simulink model "R2"  (R2016a)
settings: Solver=VariableStepAuto  StartTime=0.0  StopTime=15  MaxStep=0.01  RelTol=1e-3
values from neighbouring files (symbols this model uses):
  A = [0, 1, 0, 0 ... (first row only)    [Data.m]
  B = [0 ; 0; 0; 1]    [Data.m]
  K = acker (A, B, P)    [Data.m]
  l = 50    [Data.m]
settings Model: Creator=NAD  LastModifiedBy=NAD

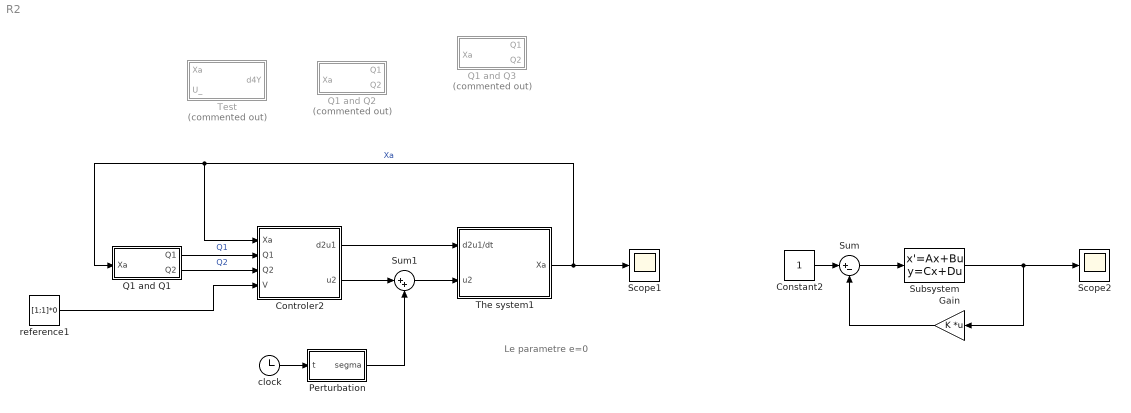
== system R2 ==
  note: Le parametre e=0
  Constant2 : Constant
  Controler2 : MATLAB Function  TreatAsAtomicUnit=on
  Gain : Gain  Gain=K  Multiplication=Matrix(K*u) (u vector)
  Perturbation : MATLAB Function  TreatAsAtomicUnit=on
  Q1 and Q1 : Subsystem
  Q1 and Q2 : Subsystem  Commented=on
  Q1 and Q3 : Subsystem  Commented=on
  Scope1 : Scope
  Scope2 : Scope
  Subsystem : StateSpace  A=A  B=B  C=eye(4)  D=[0 0 0 0 ]'  X0=0
  Sum : Sum  Inputs=|+-
  Sum1 : Sum  Inputs=|++
  Test : MATLAB Function  Commented=on  TreatAsAtomicUnit=on
  The system1 : Subsystem
  clock : Clock
  reference1 : Constant  Value=[1;1]*0
  wires:
  Subsystem/1 -> Scope2/1, Gain/1
  Sum/1 -> Subsystem/1
  Gain/1 -> Sum/2
  Constant2/1 -> Sum/1
  The system1/1(Xa) -> Q1 and Q1/1(Xa), Controler2/1(Xa), Scope1/1  "Xa"
  reference1/1 -> Controler2/4(V)
  Q1 and Q1/1(Q1) -> Controler2/2(Q1)  "Q1"
  Q1 and Q1/2(Q2) -> Controler2/3(Q2)  "Q2"
  Controler2/1(d2u1) -> The system1/1(d2u1/dt)
  Controler2/2(u2) -> Sum1/1
  Sum1/1 -> The system1/2(u2)
  clock/1 -> Perturbation/1(t)
  Perturbation/1(segma) -> Sum1/2

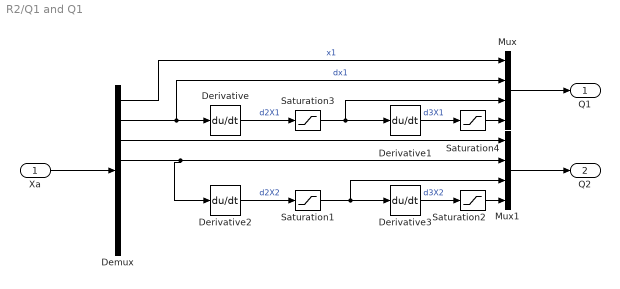
== system R2/Q1 and Q1 ==
  Xa : Inport
  Demux : Demux  Outputs=8
  Derivative{,1..3} (4 alike) : Derivative
  Mux : Mux
  Mux1 : Mux
  Saturation{1..4} (4 alike) : Saturate  UpperLimit=l  LowerLimit=-l  ZeroCross=off
  Q1 : Outport
  Q2 : Outport  Port=2
  wires:
  Mux1/1 -> Q2/1
  Mux/1 -> Q1/1
  Demux/3 -> Mux1/1
  Derivative1/1 -> Saturation4/1  "d3X1"
  Demux/1 -> Mux/1  "x1"
  Xa/1 -> Demux/1
  Derivative3/1 -> Saturation2/1  "d3X2"
  Demux/4 -> Derivative2/1, Mux1/2
  Demux/2 -> Mux/2, Derivative/1  "dx1"
  Saturation4/1 -> Mux/4
  Saturation2/1 -> Mux1/4
  Derivative2/1 -> Saturation1/1  "d2X2"
  Derivative/1 -> Saturation3/1  "d2X1"
  Saturation3/1 -> Mux/3, Derivative1/1
  Saturation1/1 -> Derivative3/1, Mux1/3

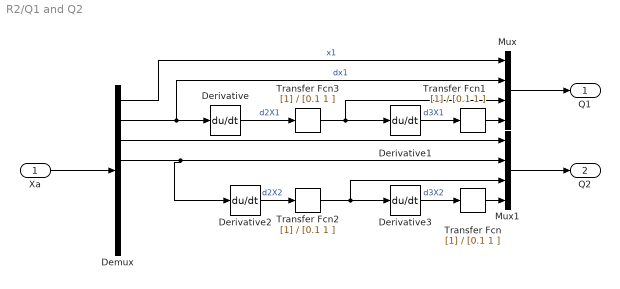
== system R2/Q1 and Q2 ==
  Xa : Inport
  Demux : Demux  Outputs=8
  Derivative{,1..3} (4 alike) : Derivative
  Mux : Mux
  Mux1 : Mux
  Transfer Fcn{,1..3} (4 alike) : TransferFcn  Denominator=[0.1 1 ]
  Q1 : Outport
  Q2 : Outport  Port=2
  wires:
  Mux1/1 -> Q2/1
  Mux/1 -> Q1/1
  Demux/3 -> Mux1/1
  Derivative1/1 -> Transfer Fcn1/1  "d3X1"
  Demux/1 -> Mux/1  "x1"
  Xa/1 -> Demux/1
  Derivative3/1 -> Transfer Fcn/1  "d3X2"
  Demux/4 -> Derivative2/1, Mux1/2
  Demux/2 -> Mux/2, Derivative/1  "dx1"
  Transfer Fcn1/1 -> Mux/4
  Transfer Fcn/1 -> Mux1/4
  Derivative2/1 -> Transfer Fcn2/1  "d2X2"
  Derivative/1 -> Transfer Fcn3/1  "d2X1"
  Transfer Fcn3/1 -> Mux/3, Derivative1/1
  Transfer Fcn2/1 -> Derivative3/1, Mux1/3

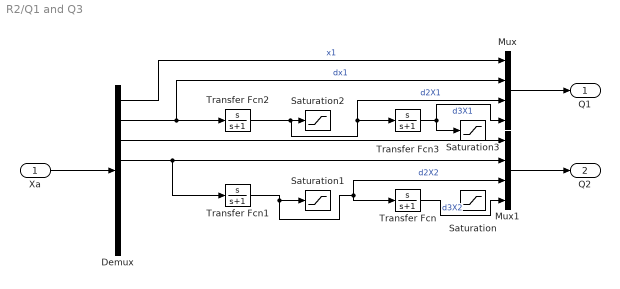
== system R2/Q1 and Q3 ==
  Xa : Inport
  Demux : Demux  Outputs=8
  Mux : Mux
  Mux1 : Mux
  Saturation{,1..3} (4 alike) : Saturate  UpperLimit=5  LowerLimit=-5  ZeroCross=off
  Transfer Fcn{,1..3} (4 alike) : TransferFcn  Numerator=[1 0]  Denominator=[1 1]
  Q1 : Outport
  Q2 : Outport  Port=2
  wires:
  Transfer Fcn/1 -> Mux1/4  "d3X2"
  Mux1/1 -> Q2/1
  Mux/1 -> Q1/1
  Demux/3 -> Mux1/1
  Transfer Fcn3/1 -> Saturation3/1, Mux/4  "d3X1"
  Demux/1 -> Mux/1  "x1"
  Xa/1 -> Demux/1
  Transfer Fcn1/1 -> Saturation1/1, Mux1/3, Transfer Fcn/1  "d2X2"
  Demux/4 -> Mux1/2, Transfer Fcn1/1
  Transfer Fcn2/1 -> Saturation2/1, Mux/3, Transfer Fcn3/1  "d2X1"
  Demux/2 -> Mux/2, Transfer Fcn2/1  "dx1"

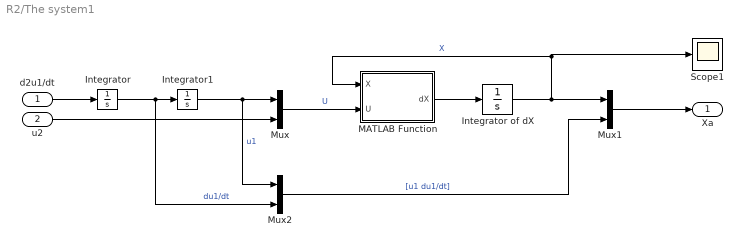
== system R2/The system1 ==
  d2u1/dt : Inport
  u2 : Inport  Port=2
  Integrator : Integrator
  Integrator of dX : Integrator  InitialCondition=[1 1 1 1 1 1]
  Integrator1 : Integrator  InitialCondition=0.1
  MATLAB Function : MATLAB Function  TreatAsAtomicUnit=on
  Mux : Mux  Inputs=2
  Mux1 : Mux  Inputs=2
  Mux2 : Mux  Inputs=2
  Scope1 : Scope
  Xa : Outport
  wires:
  MATLAB Function/1(dX) -> Integrator of dX/1
  Integrator of dX/1 -> MATLAB Function/1(X), Scope1/1, Mux1/1  "X"
  Integrator/1 -> Mux2/2, Integrator1/1  "du1/dt"
  d2u1/dt/1 -> Integrator/1
  Integrator1/1 -> Mux2/1, Mux/1  "u1"
  u2/1 -> Mux/2
  Mux/1 -> MATLAB Function/2(U)  "U"
  Mux1/1 -> Xa/1
  Mux2/1 -> Mux1/2  "[u1 du1/dt]"

== matlab function R2/The system1/MATLAB Function ==
  data: X input size=6; dX output size=6; U input size=2
function dX = fcn(X,U)
%% Definion of parameters:
x1 = X(1);
x2 = X(2);
x3 = X(3);
x4 = X(4);
x5 = X(5);
x6 = X(6);

u1 = U(1);
u2 = U(2);

e = 1e-3*0;
%% The system:
dX = [x2
    -sin(x5)*u1 + e*cos(x5)*u2
    x4
    cos(x5)*u1 + e*sin(x5)*u2-1
    x6
    u2 ];

== matlab function R2/Controler2 ==
  data: Xa input size=8; Q1 input size=4; Q2 input size=4; d2u1 output size=1; V input size=2; u2 output size=1
function [d2u1,u2]= fcn(Xa,Q1,Q2,V)
%% Definion of parameters:
x1 = Xa(1);
x2 = Xa(2);
x3 = Xa(3);
x4 = Xa(4);
x5 = Xa(5);
x6 = Xa(6);
x7 = Xa(7);
x8 = Xa(8);
e = 1e-3;

%% The feedback:
 K = [16    32    24     8]*100; % see the R2
 W1 = -K*Q1;
 W2 = -K*Q2;
 
 W = [W1;W2] + V;
%% The cintrol U_= [d2U1/dt; U2]: 
alpha_ = [-2*x8*cos(x5)*x6+x7*sin(x5)*x6^2
          -2*x8*sin(x5)*x6-x7*cos(x5)*x6^2];
beta_ = [-sin(x5) , -x7*cos(x5)
       cos(x5) , -x7*sin(x5)];

U_= beta_\(W-alpha_);
d2u1 = U_(1);
u2 = U_(2);

== matlab function R2/Perturbation ==
  data: t input size=1; segma output size=1
function segma= pertrubation(t)
segma = 200;
if (t>5)
    segma = 200*sin(10*t)*0;
end
end

== matlab function R2/Test ==
  data: Xa input size=8; U_ input size=2; d4Y output size=2
function d4Y = fcn(Xa, U_)
%% Definion of parameters:
x1 = Xa(1);
x2 = Xa(2);
x3 = Xa(3);
x4 = Xa(4);
x5 = Xa(5);
x6 = Xa(6);
x7 = Xa(7);
x8 = Xa(8);

%%
% Y1 = x1;
% dY1 = x2;
% d2Y1 = -x7*sin(x5);
% d3Y1 = -x7*cos(x5)*x6-x8*sin(x5);
% -x7*sin(x5)*x6+x8*cos

%% The cintrol U_= [d2U1/dt; U2]: 
alpha_ = [-2*x8*cos(x5)*x6+x7*sin(x5)*x6^2
          -2*x8*sin(x5)*x6-x7*cos(x5)*x6^2];
beta_ = [-sin(x5) , -x7*cos(x5)
       cos(x5) , -x7*sin(x5)];

d4Y = alpha_ + beta_*U_ ;
% Q1 = [dY1;d2Y1;d3Y1;d4Y(1)];
